simulink model "GFLIB_Acos_BAM_F32"  (Simulink 8.3)
settings: Solver=ode45  StartTime=0.0  StopTime=10.0  RelTol=1e-3
settings Model: Creator=RE004C  LastModifiedBy=B17364
settings OptimizationCC: ExpressionDepthLimit=2147483647
settings DebuggingCC: FcnCallInpInsideContextMsg=UseLocalSettings  StrictBusMsg=Warning
settings HardwareCC: ProdLargestAtomicInteger=Long  ProdLargestAtomicFloat=Double  ProdIntDivRoundTo=Zero  ProdEndianess=BigEndian  ProdHWDeviceType=Freescale->32-bit PowerPC

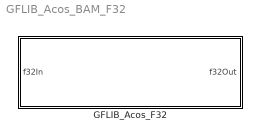
== system GFLIB_Acos_BAM_F32 ==
  GFLIB_Acos_F32 : Subsystem  mask(GFLIB_Acos_F32){}
      mask help: Bit accurate model of GFLIB_Acos function, which computes the acos(fltIn) using the 4th order Taylor polynomial approximation.
      mask init:
      | pos = get_param(gcb, 'Position');width = pos(3) - pos(1); height = pos(4) - pos(2);tX=width/2;tY=height*0.9;
      mask Display: color('black');port_label('input',1,'f32In');port_label('output',1,'f32Out');color('black');disp('GFLIB_Acos_F32');color('blue');text(tX,tY, 'BAM', 'horizontalAlignment', 'center');

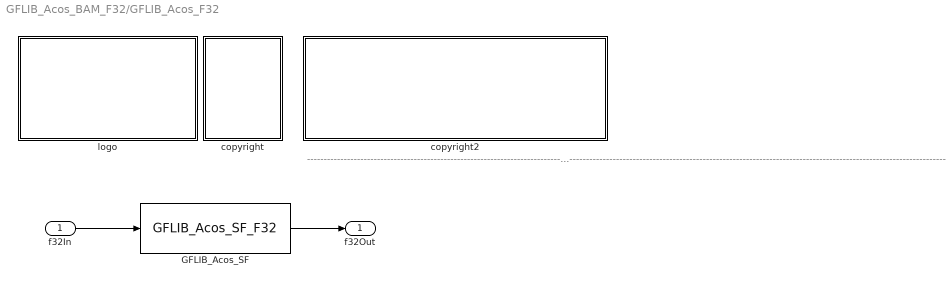
== system GFLIB_Acos_BAM_F32/GFLIB_Acos_F32 ==
  note: ---------------------------------------------------------------------------------------------------------------------------------------------------------------------------------------------------
  f32In : Inport
  GFLIB_Acos_SF : S-Function  FunctionName=GFLIB_Acos_SF_F32  EnableBusSupport=off
  copyright : Subsystem
      mask Display:
      | text(10,90,'FILE:');text(10,75,'DESRIPTION:')
      | text(10,60,'COPYRIGHT:')
      | text(10,45,'VERSION:')
      | text(10,30,'DATE:')
  copyright2 : Subsystem
      mask Display:
      | text(10,90,'GFLIB_Acos_BAM_F32.mdl');text(10,75,'Inverse cosine transformation');text(10,60,'Freescale')
      | text(10,45,'0.1');text(10,30,'31-Aug-2011');
  logo : Subsystem
      mask Display: image(imread('logo.jpg'))
  f32Out : Outport
  wires:
  f32In/1 -> GFLIB_Acos_SF/1
  GFLIB_Acos_SF/1 -> f32Out/1

== system GFLIB_Acos_BAM_F32/GFLIB_Acos_F32/copyright ==

== system GFLIB_Acos_BAM_F32/GFLIB_Acos_F32/copyright2 ==

== system GFLIB_Acos_BAM_F32/GFLIB_Acos_F32/logo ==
